simulink model "KoPilot_Demo"  (R2021b)
settings: Solver=VariableStepAuto  StartTime=0.0  StopTime=10.0  RelTol=1e-3
settings Model: Creator=ZW  LastModifiedBy=ZW

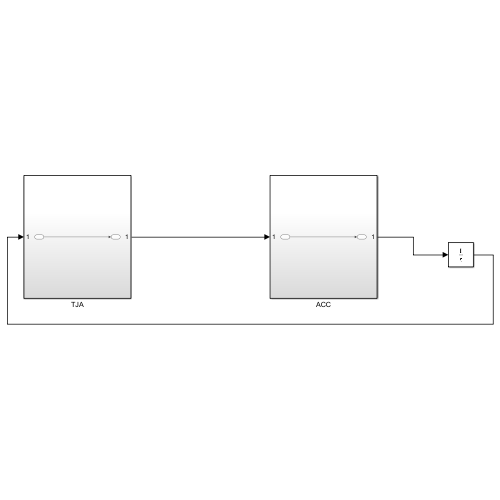
[thumbnail: Simulink's stored preview of the top-level diagram]
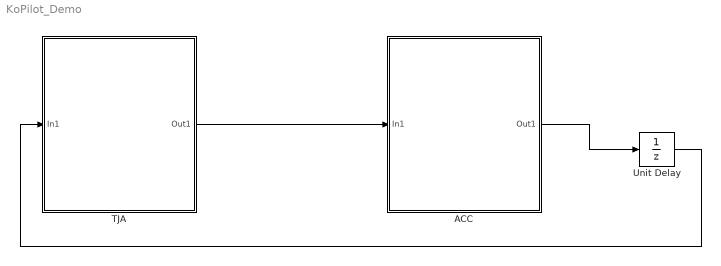
== system KoPilot_Demo ==
  ACC : Subsystem
  TJA : Subsystem
  Unit Delay : UnitDelay  SampleTime=-1  HasFrameUpgradeWarning=on
  wires:
  TJA/1(Out1) -> ACC/1(In1)
  ACC/1(Out1) -> Unit Delay/1
  Unit Delay/1 -> TJA/1(In1)

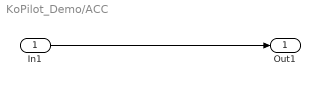
== system KoPilot_Demo/ACC ==
  In1 : Inport
  Out1 : Outport
  wires:
  In1/1 -> Out1/1

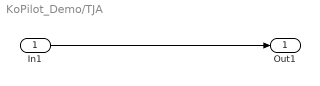
== system KoPilot_Demo/TJA ==
  In1 : Inport
  Out1 : Outport
  wires:
  In1/1 -> Out1/1
